simulink model "Lab3_Q1"  (R2020b)
settings: Solver=VariableStepAuto  StartTime=0.0  StopTime=200.0  RelTol=1e-3
settings Model: Creator=kushagrakhatwani  LastModifiedBy=kushagrakhatwani

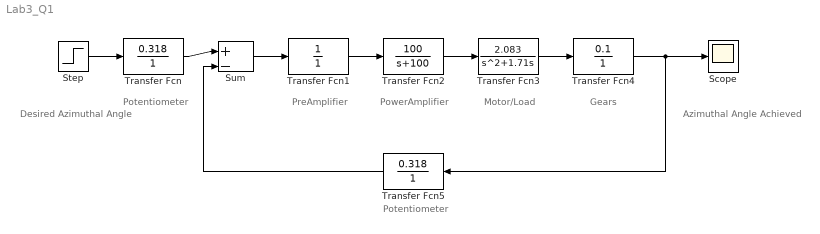
== system Lab3_Q1 ==
  note: Azimuthal Angle Achieved
  note: Desired Azimuthal Angle
  note: Gears
  note: Motor/Load
  note: PowerAmplifier
  note: PreAmplifier
  note: Potentiometer
  note: Potentiometer
  Scope : Scope
  Step : Step  Time=0  SampleTime=0
  Sum : Sum  Inputs=|+-
  Transfer Fcn : TransferFcn  Numerator=[0.318]  Denominator=[1]
  Transfer Fcn1 : TransferFcn  Denominator=[1]
  Transfer Fcn2 : TransferFcn  Numerator=[100]  Denominator=[1 100]
  Transfer Fcn3 : TransferFcn  Numerator=[2.083]  Denominator=[1 1.71 0]
  Transfer Fcn4 : TransferFcn  Numerator=[0.1]  Denominator=[1]
  Transfer Fcn5 : TransferFcn  Numerator=[0.318]  Denominator=[1]
  wires:
  Step/1 -> Transfer Fcn/1
  Transfer Fcn/1 -> Sum/1
  Sum/1 -> Transfer Fcn1/1
  Transfer Fcn1/1 -> Transfer Fcn2/1
  Transfer Fcn2/1 -> Transfer Fcn3/1
  Transfer Fcn3/1 -> Transfer Fcn4/1
  Transfer Fcn5/1 -> Sum/2
  Transfer Fcn4/1 -> Transfer Fcn5/1, Scope/1
